simulink model "dbx_control_v1_00"  (R2015a)
settings: Solver=FixedStepDiscrete  SolverMode=SingleTasking  StartTime=0.0  StopTime=20  FixedStep=T_ctrl  RelTol=1e-3
undefined symbols (not defined in the file): A_l_max_x, A_M, A_z_max, CG, epsilon, Flaps_ang_deg, g, h_1, h_2, h_3, Hover_eta_23, Hover_throtle_1, Hover_throtle_23, I_BAC, L_M, m, Roll_pich_sens, Rotation_sign, Servo_calib, T_ctrl, v_i0, Yaw_sens
libraries: DBX_model x29, DBX_Control_lib x22, simulink x10, DBX_Control x3
(part 1 of 3)
settings Model: ExtModeTrigDuration=5000  TunableVars=Flaps_ang_deg,Roll_pich_sens,Throtle_sens,Yaw_sens,p_K_b,p_tau,phi_K_b,phi_f_i,phi_tau,psi_K_b,psi_f_i,psi_tau,q_K_b,q_tau,r_K_b,r_tau,theta_K_b,theta_f_i,theta_tau  TunableVarsStorageClass=Auto,Auto,Auto,Auto,Auto,Auto,Auto,Auto,Auto,Auto,Auto,Auto,Auto,Auto,Auto,Auto,Auto,Auto,Auto  TunableVarsTypeQualifier=,,,,,,,,,,,,,,,,,,  Creator=DavidTorres  LastModifiedBy=David
settings DataIOCC: LimitDataPoints=off  SaveOutput=off  SignalLogging=off  DSMLogging=off  VisualizeSimOutput=off  SaveTime=off
settings OptimizationCC: InlineParams=on  UseDivisionForNetSlopeComputation=on  DefaultUnderspecifiedDataType=single  UseSpecifiedMinMax=on  EfficientFloat2IntCast=on  OptimizeModelRefInitCode=on  MaxStackSize=64  SimCompilerOptimization=on
settings DebuggingCC: SaveWithParameterizedLinksMsg=none  IntegerOverflowMsg=error  StrictBusMsg=ErrorOnBusTreatedAsVector  IntegerSaturationMsg=error
settings HardwareCC: ProdLargestAtomicInteger=Long  ProdLargestAtomicFloat=Double  ProdIntDivRoundTo=Zero  ProdEndianess=LittleEndian  ProdHWDeviceType=Generic->32-bit x86 compatible  TargetLongLongMode=on  TargetIntDivRoundTo=Zero  TargetEndianess=LittleEndian  TargetHWDeviceType=MATLAB Host  ProdEqTarget=off
settings ModelReferenceCC: ModelReferenceNumInstancesAllowed=Single  ModelReferencePassRootInputsByReference=off
settings RTWCC: SystemTargetFile=ert.tlc  GenCodeOnly=on  TemplateMakefile=ert_default_tmf  Description=Embedded Coder  BuildConfiguration=Faster Runs
settings CodeAppCC: IgnoreCustomStorageClasses=off
settings ERTTargetCC: GenerateSampleERTMain=off  ParMdlRefBuildCompliant=on  CompOptLevelCompliant=on  ConcurrentExecutionCompliant=on  ERTFirstTimeCompliant=on  SupportNonFinite=off  SupportComplex=off  SupportContinuousTime=off  ModelStepFunctionPrototypeControlCompliant=on  CPPClassGenCompliant=on  InlinedParameterPlacement=Hierarchical  ERTCustomFileTemplate=example_file_process.tlc

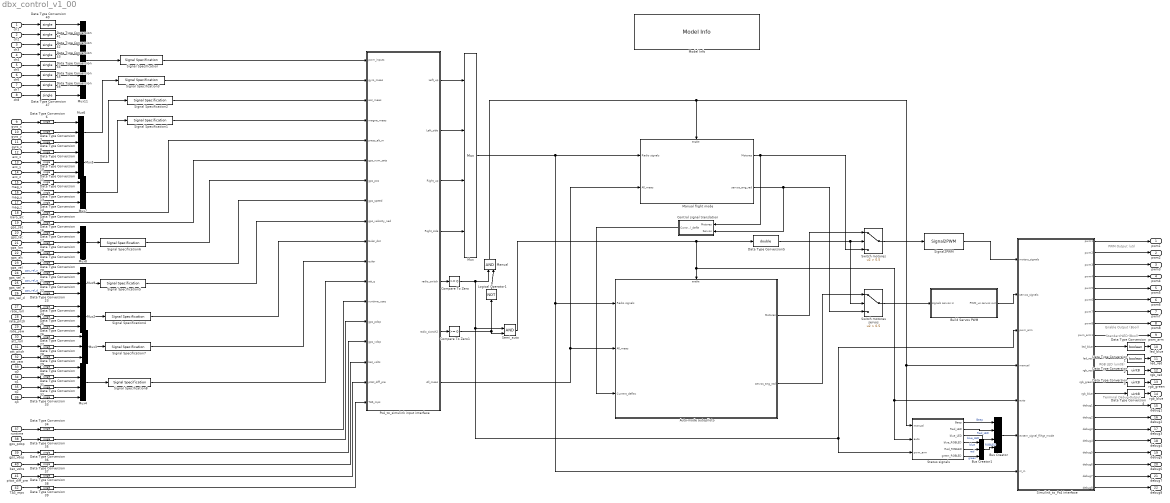
== system dbx_control_v1_00 ==
  note: Terminal Debug Output
  note: RGB LED (uint8)
  note: Standard LED (Bool)
  note: PWM Output (uS)
  note: Enable Output (Bool)
  ch1 : Inport  OutDataTypeStr=double  PortDimensions=[1,1]  SampleTime=T_ctrl
  ch2 : Inport  Port=2  OutDataTypeStr=double  PortDimensions=[1,1]  SampleTime=T_ctrl
  ch3 : Inport  Port=3  OutDataTypeStr=double  PortDimensions=[1,1]  SampleTime=T_ctrl
  ch4 : Inport  Port=4  OutDataTypeStr=double  PortDimensions=[1,1]  SampleTime=T_ctrl
  ch5 : Inport  Port=5  OutDataTypeStr=double  PortDimensions=[1,1]  SampleTime=T_ctrl
  ch6 : Inport  Port=6  OutDataTypeStr=double  PortDimensions=[1,1]  SampleTime=T_ctrl
  ch7 : Inport  Port=7  OutDataTypeStr=double  PortDimensions=[1,1]  SampleTime=T_ctrl
  ch8 : Inport  Port=8  OutDataTypeStr=double  PortDimensions=[1,1]  SampleTime=T_ctrl
  gyro_x : Inport  Port=9  OutDataTypeStr=double  PortDimensions=[1,1]  SampleTime=T_ctrl
  gyro_y : Inport  Port=10  OutDataTypeStr=double  PortDimensions=[1,1]  SampleTime=T_ctrl
  gyro_z : Inport  Port=11  OutDataTypeStr=double  PortDimensions=[1,1]  SampleTime=T_ctrl
  acc_x : Inport  Port=12  OutDataTypeStr=double  PortDimensions=[1,1]  SampleTime=T_ctrl
  acc_y : Inport  Port=13  OutDataTypeStr=double  PortDimensions=[1,1]  SampleTime=T_ctrl
  acc_z : Inport  Port=14  OutDataTypeStr=double  PortDimensions=[1,1]  SampleTime=T_ctrl
  mag_x : Inport  Port=15  OutDataTypeStr=double  PortDimensions=[1,1]  SampleTime=T_ctrl
  mag_y : Inport  Port=16  OutDataTypeStr=double  PortDimensions=[1,1]  SampleTime=T_ctrl
  mag_z : Inport  Port=17  OutDataTypeStr=double  PortDimensions=[1,1]  SampleTime=T_ctrl
  baro_alt : Inport  Port=18  OutDataTypeStr=double  PortDimensions=[1,1]  SampleTime=T_ctrl
  gps_sat : Inport  Port=19  OutDataTypeStr=double  PortDimensions=[1,1]  SampleTime=T_ctrl
  gps_lat : Inport  Port=20  OutDataTypeStr=double  PortDimensions=[1,1]  SampleTime=T_ctrl
  gps_lon : Inport  Port=21  OutDataTypeStr=double  PortDimensions=[1,1]  SampleTime=T_ctrl
  gps_alt : Inport  Port=22  OutDataTypeStr=double  PortDimensions=[1,1]  SampleTime=T_ctrl
  gps_vel : Inport  Port=23  OutDataTypeStr=double  PortDimensions=[1,1]  SampleTime=T_ctrl
  gps_vel_n : Inport  Port=24  OutDataTypeStr=double  PortDimensions=[1,1]  SampleTime=T_ctrl
  gps_vel_e : Inport  Port=25  OutDataTypeStr=double  PortDimensions=[1,1]  SampleTime=T_ctrl
  gps_vel_d : Inport  Port=26  OutDataTypeStr=double  PortDimensions=[1,1]  SampleTime=T_ctrl
  rate_roll : Inport  Port=27  OutDataTypeStr=double  PortDimensions=[1,1]  SampleTime=T_ctrl
  rate_pitch : Inport  Port=28  OutDataTypeStr=double  PortDimensions=[1,1]  SampleTime=T_ctrl
  rate_yaw : Inport  Port=29  OutDataTypeStr=double  PortDimensions=[1,1]  SampleTime=T_ctrl
  att_roll : Inport  Port=30  OutDataTypeStr=double  PortDimensions=[1,1]  SampleTime=T_ctrl
  att_pitch : Inport  Port=31  OutDataTypeStr=double  PortDimensions=[1,1]  SampleTime=T_ctrl
  att_yaw : Inport  Port=32  OutDataTypeStr=double  PortDimensions=[1,1]  SampleTime=T_ctrl
  q0 : Inport  Port=33  OutDataTypeStr=double  PortDimensions=[1,1]  SampleTime=T_ctrl
  q1 : Inport  Port=34  OutDataTypeStr=double  PortDimensions=[1,1]  SampleTime=T_ctrl
  q2 : Inport  Port=35  OutDataTypeStr=double  PortDimensions=[1,1]  SampleTime=T_ctrl
  q3 : Inport  Port=36  OutDataTypeStr=double  PortDimensions=[1,1]  SampleTime=T_ctrl
  runtime : Inport  Port=37  OutDataTypeStr=double  PortDimensions=[1,1]  SampleTime=T_ctrl
  gps_pdop : Inport  Port=38  OutDataTypeStr=double  PortDimensions=[1,1]  SampleTime=T_ctrl
  gps_vdop : Inport  Port=39  OutDataTypeStr=double  PortDimensions=[1,1]  SampleTime=T_ctrl
  bat_volts : Inport  Port=40  OutDataTypeStr=double  PortDimensions=[1,1]  SampleTime=T_ctrl
  pitot_diff_pre : Inport  Port=41  OutDataTypeStr=double  SampleTime=T_ctrl
  TAS_mps : Inport  Port=42  OutDataTypeStr=double  SampleTime=T_ctrl
  Auto-mode autopiloto : Subsystem  TreatAsAtomicUnit=on
  Build Servos PWM : Subsystem  TreatAsAtomicUnit=on
  Bus Creator : BusCreator
  Bus Creator1 : BusCreator  Inputs=3
  Compare To Zero : simulink/Logic and Bit Operations/Compare To Zero  relop=>=  OutDataTypeStr=boolean
  Compare To Zero1 : simulink/Logic and Bit Operations/Compare To Zero  relop=>=  OutDataTypeStr=boolean
  Control signal translation : Subsystem  TreatAsAtomicUnit=on
  Data Type Conversion : DataTypeConversion  OutDataTypeStr=boolean
  Data Type Conversion1 : DataTypeConversion  OutDataTypeStr=boolean
  Data Type Conversion{6..47} (42 alike) : DataTypeConversion  OutDataTypeStr=single
  Data Type Conversion2 : DataTypeConversion  OutDataTypeStr=uint8
  Data Type Conversion3 : DataTypeConversion  OutDataTypeStr=uint8
  Data Type Conversion4 : DataTypeConversion  OutDataTypeStr=uint8
  Data Type Conversion5 : DataTypeConversion  OutDataTypeStr=double
  Logical Operator1 : Logic  Operator=NOT  IconShape=distinctive  AllPortsSameDT=off  OutDataTypeStr=boolean
  Manual : Logic  IconShape=distinctive  AllPortsSameDT=off  OutDataTypeStr=boolean
  Manual flight mode : Subsystem  TreatAsAtomicUnit=on
  Model Info : simulink/Model-Wide Utilities/Model Info  Frame=on  DisplayStringWithTags=|  HorizontalTextAlignment=Center  LeftAlignmentValue=0.5  SourceBlockDiagram=dbx_control_v1_00  TagMaxNumber=20
      | Model Info
      | 
      | Creado por %<Creator>
      | Modificado el %<LastModificationDate> por %<LastModifiedBy>
      | Version %<ModelVersion>
  Mux : Mux
  Mux11 : Mux  Inputs=8
  Mux{2..3,5..9} (7 alike) : Mux  Inputs=3
  Mux4 : Mux
  Px4_to_simulink input interface : Subsystem
  Semi_auto : Logic  IconShape=distinctive  AllPortsSameDT=off  OutDataTypeStr=boolean
  Signal Specification : SignalSpecification  OutDataTypeStr=single  Dimensions=[8,1]
  Signal Specification{1..7} (7 alike) : SignalSpecification  OutDataTypeStr=single  Dimensions=[3,1]
  Signal Specification8 : SignalSpecification  OutDataTypeStr=single  Dimensions=[4,1]
  Signal2PWM : DBX_model/Signal2PWM  b=1  d=0  a=1900  c=1100
  Simulink_to_Px4 interface : Subsystem
  Status signals : Subsystem  TreatAsAtomicUnit=on
  Switch motores : Switch  Criteria=u2 > Threshold  Threshold=0.5
  Switch motores servos : Switch  Criteria=u2 > Threshold  Threshold=0.5
  pwm1 : Outport  PortDimensions=[1,1]
  pwm2 : Outport  Port=2  PortDimensions=[1,1]
  pwm3 : Outport  Port=3  PortDimensions=[1,1]
  pwm4 : Outport  Port=4  PortDimensions=[1,1]
  pwm5 : Outport  Port=5  PortDimensions=[1,1]
  pwm6 : Outport  Port=6  PortDimensions=[1,1]
  pwm7 : Outport  Port=7  PortDimensions=[1,1]
  pwm8 : Outport  Port=8  PortDimensions=[1,1]
  pwm_arm : Outport  Port=9  PortDimensions=[1,1]
  led_blue : Outport  Port=10  OutDataTypeStr=boolean  PortDimensions=[1,1]
  led_red : Outport  Port=11  OutDataTypeStr=boolean  PortDimensions=[1,1]
  rgb_red : Outport  Port=12  OutDataTypeStr=uint8  PortDimensions=[1,1]
  rgb_green : Outport  Port=13  OutDataTypeStr=uint8  PortDimensions=[1,1]
  rgb_blue : Outport  Port=14  OutDataTypeStr=uint8  PortDimensions=[1,1]
  debug1 : Outport  Port=15  PortDimensions=[1,1]
  debug2 : Outport  Port=16  PortDimensions=[1,1]
  debug3 : Outport  Port=17  PortDimensions=[1,1]
  debug4 : Outport  Port=18  PortDimensions=[1,1]
  debug5 : Outport  Port=19  PortDimensions=[1,1]
  debug6 : Outport  Port=20  PortDimensions=[1,1]
  debug7 : Outport  Port=21  PortDimensions=[1,1]
  debug8 : Outport  Port=22  PortDimensions=[1,1]
  wires:
  Switch motores/1 -> Signal2PWM/1
  Switch motores servos/1 -> Build Servos PWM/1(signals servos in)
  Status signals/1(Beep) -> Bus Creator/1  "Beep"
  Status signals/2(Red_LED) -> Bus Creator/2  "Red_LED"
  Status signals/3(blue_LED) -> Bus Creator/3  "blue_LED"
  Status signals/4(blue_RGBLED) -> Bus Creator1/1  "blue"
  Status signals/5(Red_RGBLED) -> Bus Creator1/2  "red"
  Status signals/6(green_RGBLED) -> Bus Creator1/3  "green"
  Bus Creator1/1 -> Bus Creator/4  "RGBLED"
  Simulink_to_Px4 interface/1(pwm1) -> pwm1/1
  Simulink_to_Px4 interface/2(pwm2) -> pwm2/1
  Simulink_to_Px4 interface/3(pwm3) -> pwm3/1
  Simulink_to_Px4 interface/4(pwm4) -> pwm4/1
  Simulink_to_Px4 interface/5(pwm5) -> pwm5/1
  Simulink_to_Px4 interface/6(pwm6) -> pwm6/1
  Simulink_to_Px4 interface/7(pwm7) -> pwm7/1
  Simulink_to_Px4 interface/8(pwm8) -> pwm8/1
  Simulink_to_Px4 interface/10(led_blue) -> Data Type Conversion/1
  Simulink_to_Px4 interface/11(led_red) -> Data Type Conversion1/1
  Simulink_to_Px4 interface/15(debug1) -> debug1/1
  Simulink_to_Px4 interface/17(debug3) -> debug3/1
  Simulink_to_Px4 interface/18(debug4) -> debug4/1
  Simulink_to_Px4 interface/9(pwm_arm1) -> pwm_arm/1
  Simulink_to_Px4 interface/12(rgb_red) -> Data Type Conversion2/1
  Simulink_to_Px4 interface/13(rgb_green) -> Data Type Conversion3/1
  Simulink_to_Px4 interface/14(rgb_blue) -> Data Type Conversion4/1
  Simulink_to_Px4 interface/20(debug6) -> debug6/1
  Simulink_to_Px4 interface/21(debug7) -> debug7/1
  Simulink_to_Px4 interface/22(debug8) -> debug8/1
  Simulink_to_Px4 interface/19(debug5) -> debug5/1
  Data Type Conversion/1 -> led_blue/1
  Data Type Conversion1/1 -> led_red/1
  Data Type Conversion2/1 -> rgb_red/1
  Data Type Conversion3/1 -> rgb_green/1
  Data Type Conversion4/1 -> rgb_blue/1
  Simulink_to_Px4 interface/16(debug2) -> debug2/1
  Signal2PWM/1 -> Simulink_to_Px4 interface/1(motors_signals)
  Build Servos PWM/1(PWM_us servos out) -> Simulink_to_Px4 interface/2(servos_signals)
  Bus Creator/1 -> Simulink_to_Px4 interface/6(extern_signal_flihgt_mode)
  baro_alt/1 -> Data Type Conversion15/1
  gyro_z/1 -> Data Type Conversion8/1
  gyro_y/1 -> Data Type Conversion7/1
  gyro_x/1 -> Data Type Conversion6/1
  acc_z/1 -> Data Type Conversion11/1
  acc_y/1 -> Data Type Conversion10/1
  acc_x/1 -> Data Type Conversion9/1
  mag_x/1 -> Data Type Conversion12/1
  mag_y/1 -> Data Type Conversion13/1
  mag_z/1 -> Data Type Conversion14/1
  ch1/1 -> Data Type Conversion40/1
  ch2/1 -> Data Type Conversion41/1
  ch3/1 -> Data Type Conversion42/1
  ch4/1 -> Data Type Conversion43/1
  ch5/1 -> Data Type Conversion44/1
  ch6/1 -> Data Type Conversion45/1
  runtime/1 -> Data Type Conversion34/1
  ch7/1 -> Data Type Conversion46/1
  ch8/1 -> Data Type Conversion47/1
  att_roll/1 -> Data Type Conversion27/1
  att_pitch/1 -> Data Type Conversion28/1
  att_yaw/1 -> Data Type Conversion29/1
  q0/1 -> Data Type Conversion30/1
  q1/1 -> Data Type Conversion31/1
  q2/1 -> Data Type Conversion32/1
  q3/1 -> Data Type Conversion33/1
  rate_roll/1 -> Data Type Conversion24/1
  rate_pitch/1 -> Data Type Conversion25/1
  rate_yaw/1 -> Data Type Conversion26/1
  gps_vel_n/1 -> Data Type Conversion21/1  "gps_vel_n"
  gps_vel_e/1 -> Data Type Conversion22/1  "gps_vel_e"
  gps_vel_d/1 -> Data Type Conversion23/1  "gps_vel_d"
  gps_lat/1 -> Data Type Conversion17/1
  gps_lon/1 -> Data Type Conversion18/1
  gps_alt/1 -> Data Type Conversion19/1
  gps_vel/1 -> Data Type Conversion20/1
  gps_sat/1 -> Data Type Conversion16/1
  Mux2/1 -> Signal Specification4/1
  Mux3/1 -> Signal Specification7/1
  Mux4/1 -> Signal Specification8/1
  Mux5/1 -> Signal Specification2/1
  Mux6/1 -> Signal Specification3/1
  Mux8/1 -> Signal Specification6/1
  Mux7/1 -> Signal Specification1/1
  Mux11/1 -> Signal Specification/1
  Mux9/1 -> Signal Specification5/1
  gps_pdop/1 -> Data Type Conversion35/1
  gps_vdop/1 -> Data Type Conversion36/1
  bat_volts/1 -> Data Type Conversion37/1
  Signal Specification/1 -> Px4_to_simulink input interface/1(pwm_inputs)
  Signal Specification3/1 -> Px4_to_simulink input interface/2(gyro_meas)
  Signal Specification2/1 -> Px4_to_simulink input interface/3(acc_meas)
  Signal Specification1/1 -> Px4_to_simulink input interface/4(magne_meas)
  Signal Specification6/1 -> Px4_to_simulink input interface/7(gps_pos)
  Signal Specification5/1 -> Px4_to_simulink input interface/9(gps_velocity_ned)
  Signal Specification4/1 -> Px4_to_simulink input interface/10(Euler_dot)
  Signal Specification7/1 -> Px4_to_simulink input interface/11(euler)
  Signal Specification8/1 -> Px4_to_simulink input interface/12(att_q)
  pitot_diff_pre/1 -> Data Type Conversion38/1
  Px4_to_simulink input interface/5(radio_switch) -> Compare To Zero/1
  Px4_to_simulink input interface/6(radio_siwtch2) -> Compare To Zero1/1
  Compare To Zero/1 -> Semi_auto/1, Simulink_to_Px4 interface/3(pwm_arm), Status signals/3(pwm_arm), Manual/1
  Compare To Zero1/1 -> Logical Operator1/1, Semi_auto/2
  Manual/1 -> Simulink_to_Px4 interface/4(manual), Status signals/1(manual), Manual flight mode/Enable
  Manual flight mode/2(servos_ang_rad) -> Control signal translation/2(Servos), Switch motores servos/3
  Auto-mode autopiloto/1(Motores) -> Switch motores/1
  Auto-mode autopiloto/2(servos_ang_rad) -> Switch motores servos/1
  Semi_auto/1 -> Data Type Conversion5/1, Simulink_to_Px4 interface/5(auto), Status signals/2(auto), Auto-mode autopiloto/Enable
  Data Type Conversion5/1 -> Switch motores servos/2, Switch motores/2
  Px4_to_simulink input interface/4(Right_side) -> Mux/4
  Px4_to_simulink input interface/3(Right_up) -> Mux/3
  Px4_to_simulink input interface/2(Left_side) -> Mux/2
  Px4_to_simulink input interface/1(Left_up) -> Mux/1
  Px4_to_simulink input interface/7(All_meas) -> Manual flight mode/2(All_meas), Auto-mode autopiloto/2(All_meas)
  Mux/1 -> Manual flight mode/1(Radio signals), Simulink_to_Px4 interface/7(rc_in), Auto-mode autopiloto/1(Radio signals)
  TAS_mps/1 -> Data Type Conversion39/1
  Logical Operator1/1 -> Manual/2
  Manual flight mode/1(Motores) -> Switch motores/3, Control signal translation/1(Motores)
  Control signal translation/1(Control_defle) -> Auto-mode autopiloto/3(Current_deflex)
  Data Type Conversion6/1 -> Mux6/1
  Data Type Conversion7/1 -> Mux6/2
  Data Type Conversion8/1 -> Mux6/3
  Data Type Conversion9/1 -> Mux5/1
  Data Type Conversion10/1 -> Mux5/2
  Data Type Conversion11/1 -> Mux5/3
  Data Type Conversion12/1 -> Mux7/1
  Data Type Conversion13/1 -> Mux7/2
  Data Type Conversion14/1 -> Mux7/3
  Data Type Conversion15/1 -> Px4_to_simulink input interface/5(press_alt_m)
  Data Type Conversion16/1 -> Px4_to_simulink input interface/6(gps_num_sats)
  Data Type Conversion17/1 -> Mux8/1
  Data Type Conversion18/1 -> Mux8/2
  Data Type Conversion19/1 -> Mux8/3
  Data Type Conversion20/1 -> Px4_to_simulink input interface/8(gps_speed)
  Data Type Conversion21/1 -> Mux9/1
  Data Type Conversion22/1 -> Mux9/2
  Data Type Conversion23/1 -> Mux9/3
  Data Type Conversion24/1 -> Mux2/1
  Data Type Conversion25/1 -> Mux2/2
  Data Type Conversion26/1 -> Mux2/3
  Data Type Conversion27/1 -> Mux3/1
  Data Type Conversion28/1 -> Mux3/2
  Data Type Conversion29/1 -> Mux3/3
  Data Type Conversion30/1 -> Mux4/1
  Data Type Conversion31/1 -> Mux4/2
  Data Type Conversion32/1 -> Mux4/3
  Data Type Conversion33/1 -> Mux4/4
  Data Type Conversion34/1 -> Px4_to_simulink input interface/13(runtime_usec)
  Data Type Conversion35/1 -> Px4_to_simulink input interface/14(gps_pdop)
  Data Type Conversion36/1 -> Px4_to_simulink input interface/15(gps_vdop)
  Data Type Conversion37/1 -> Px4_to_simulink input interface/16(bat_volts)
  Data Type Conversion38/1 -> Px4_to_simulink input interface/17(pitot_diff_pre)
  Data Type Conversion39/1 -> Px4_to_simulink input interface/18(TAS_mps)
  Data Type Conversion40/1 -> Mux11/1
  Data Type Conversion41/1 -> Mux11/2
  Data Type Conversion42/1 -> Mux11/3
  Data Type Conversion43/1 -> Mux11/4
  Data Type Conversion44/1 -> Mux11/5
  Data Type Conversion45/1 -> Mux11/6
  Data Type Conversion46/1 -> Mux11/7
  Data Type Conversion47/1 -> Mux11/8

== system dbx_control_v1_00/Auto-mode autopiloto ==
  Radio signals : Inport
  All_meas : Inport  Port=2
  Current_deflex : Inport  Port=3
  Enable : EnablePort  ShowOutputPort=on
  Activation bus : Subsystem  TreatAsAtomicUnit=on
  DBX advance control system : Subsystem
  Demux : Demux  Outputs=7
  Ground : Ground
  Ground1 : Ground
  Initial conditions : Subsystem  TreatAsAtomicUnit=on
  Mux : Mux  Inputs=3
  Mux1 : Mux  Inputs=7
  Mux2 : Mux  Inputs=3
  Saturation : Saturate  UpperLimit=1  LowerLimit=0
  Saturation1 : Saturate  UpperLimit=deg2rad(90)  LowerLimit=-deg2rad(90)
  Sensibilidades Radio : Subsystem  TreatAsAtomicUnit=on
  Sup2Servo Lin conversion : DBX_model/Sup2Servo Lin conversion  Gain=Servo_calib.Servo1.Pendiente_Sup_Servo  Bias=Servo_calib.Servo1.Sup_rad_0
  Sup2Servo Lin conversion1 : DBX_model/Sup2Servo Lin conversion  Gain=Servo_calib.Servo2.Pendiente_Sup_Servo  Bias=Servo_calib.Servo2.Sup_rad_0
  Sup2Servo Lin conversion2 : DBX_model/Sup2Servo Lin conversion  Gain=Servo_calib.Servo3.Pendiente_Sup_Servo  Bias=Servo_calib.Servo3.Sup_rad_0
  Sup2Servo Lin conversion3 : DBX_model/Sup2Servo Lin conversion  Gain=Servo_calib.Servo4.Pendiente_Sup_Servo  Bias=Servo_calib.Servo4.Sup_rad_0
  Sup2Servo Lin conversion4 : DBX_model/Sup2Servo Lin conversion  Gain=Servo_calib.Servo5.Pendiente_Sup_Servo  Bias=Servo_calib.Servo5.Sup_rad_0
  Sup2Servo Lin conversion5 : DBX_model/Sup2Servo Lin conversion  Gain=Servo_calib.Servo6.Pendiente_Sup_Servo  Bias=Servo_calib.Servo6.Sup_rad_0
  Sup2Servo Lin conversion6 : DBX_model/Sup2Servo Lin conversion  Gain=Servo_calib.Servo7.Pendiente_Sup_Servo  Bias=Servo_calib.Servo7.Sup_rad_0
  Terminator : Terminator
  Motores : Outport
  servos_ang_rad : Outport  Port=2
  wires:
  DBX advance control system/1(Mot_throtles) -> Saturation/1
  Saturation/1 -> Motores/1
  Mux1/1 -> Saturation1/1
  Saturation1/1 -> servos_ang_rad/1
  Sup2Servo Lin conversion/1 -> Mux1/1
  Sup2Servo Lin conversion1/1 -> Mux1/2
  Sup2Servo Lin conversion2/1 -> Mux1/3
  Sup2Servo Lin conversion3/1 -> Mux1/4
  Sup2Servo Lin conversion4/1 -> Mux1/5
  Sup2Servo Lin conversion5/1 -> Mux1/6
  Sup2Servo Lin conversion6/1 -> Mux1/7
  All_meas/1 -> Initial conditions/1(All_meas), DBX advance control system/5(All_meas)
  DBX advance control system/3(surf_angles) -> Demux/1
  Demux/1 -> Sup2Servo Lin conversion/1
  Demux/2 -> Sup2Servo Lin conversion1/1
  Demux/3 -> Sup2Servo Lin conversion2/1
  Demux/4 -> Sup2Servo Lin conversion3/1
  Demux/5 -> Sup2Servo Lin conversion4/1
  Demux/6 -> Sup2Servo Lin conversion5/1
  Demux/7 -> Sup2Servo Lin conversion6/1
  Radio signals/1 -> Sensibilidades Radio/1(Radio_in)
  Mux/1 -> DBX advance control system/3(Att_ref(rad))
  Mux2/1 -> DBX advance control system/1(Vel_ref_yaw(mps))
  Sensibilidades Radio/4(Yaw(radps)) -> DBX advance control system/4(Yaw_rate_ref(rad)), Mux/3
  Sensibilidades Radio/2(Roll(rad)) -> Mux/1
  Sensibilidades Radio/3(Vx_yaw) -> Mux2/1
  Activation bus/1(Activation bus) -> DBX advance control system/8(activation_bus)
  Enable/1 -> DBX advance control system/9(Int_reset), Activation bus/2(Activation1), Activation bus/1(Activation), Activation bus/4(Activation3), Activation bus/3(Activation2)
  Initial conditions/1(Init_cond) -> DBX advance control system/6(Init_cond)
  Current_deflex/1 -> DBX advance control system/7(Init_deflect)
  DBX advance control system/2(Control_signals) -> Terminator/1
  Ground/1 -> Mux2/3, Mux2/2
  Ground1/1 -> Mux/2
  Sensibilidades Radio/1(accz_yaw) -> DBX advance control system/2(Acc_z(mps2))

== system dbx_control_v1_00/Build Servos PWM ==
  note: Estos 4 ultimos significa que
      | los ejes de los servos deben
      | apuntar el la direccion +y
  note: Control input
      | Rango
      | Direccion rot/Dir servos
      | Rango del servo
      |
      | eta_1 (rad) (Pan arm 1)
      | -90,90
      | -1
      | 180
      |
      | eta_2 (rad) (Pan arm 2
      | -90,90
      | -1
      | 180
      |
      | eta_3 (rad) (Pan arm 3)
      | -90,90
      | 1
      | 180
      |
      | Rudervator Left (rad)
      | -90,90
      | 1
      | 180
      |
      | Rudervator Right (rad)
      | -90,90
      | 1
      | 180
      |
      | Aileron Left (rad)
      | -90,90
      | 1
      | 180
      |
      | Aielron Right (rad)
      | -90,90
      | 1
      | 180
  signals servos in : Inport
  Demux : Demux  Outputs=7
  Mux : Mux  Inputs=7
  Signal2PWM{,1..6} (7 alike) : DBX_model/Signal2PWM  b=deg2rad(90)  d=-deg2rad(90)  a=1900  c=1100
  PWM_us servos out : Outport
  wires:
  Mux/1 -> PWM_us servos out/1
  signals servos in/1 -> Demux/1
  Demux/6 -> Signal2PWM5/1
  Demux/5 -> Signal2PWM4/1
  Demux/4 -> Signal2PWM3/1
  Demux/3 -> Signal2PWM2/1
  Demux/2 -> Signal2PWM1/1
  Demux/1 -> Signal2PWM/1
  Signal2PWM/1 -> Mux/1
  Signal2PWM1/1 -> Mux/2
  Signal2PWM3/1 -> Mux/4
  Signal2PWM4/1 -> Mux/5
  Signal2PWM2/1 -> Mux/3
  Signal2PWM5/1 -> Mux/6
  Demux/7 -> Signal2PWM6/1
  Signal2PWM6/1 -> Mux/7

== system dbx_control_v1_00/Control signal translation ==
  Motores : Inport
  Servos : Inport  Port=2
  Demux : Demux  Outputs=3
  Ground{,1..4} (5 alike) : Ground
  Mux1 : Mux  Inputs=9
  Selector : Selector  InputPortWidth=7  Indices=3
  Servo2Sup Lin conversion : DBX_model/Servo2Sup Lin conversion  Gain=Servo_calib.Servo3.Pendiente_Sup_Servo  Bias=Servo_calib.Servo3.Sup_rad_0
  Control_defle : Outport
  wires:
  Mux1/1 -> Control_defle/1
  Demux/1 -> Mux1/1
  Servos/1 -> Selector/1
  Demux/2 -> Mux1/3
  Demux/3 -> Mux1/5
  Ground/1 -> Mux1/2
  Ground1/1 -> Mux1/4
  Ground2/1 -> Mux1/7
  Ground3/1 -> Mux1/8
  Ground4/1 -> Mux1/9
  Servo2Sup Lin conversion/1 -> Mux1/6
  Motores/1 -> Demux/1
  Selector/1 -> Servo2Sup Lin conversion/1

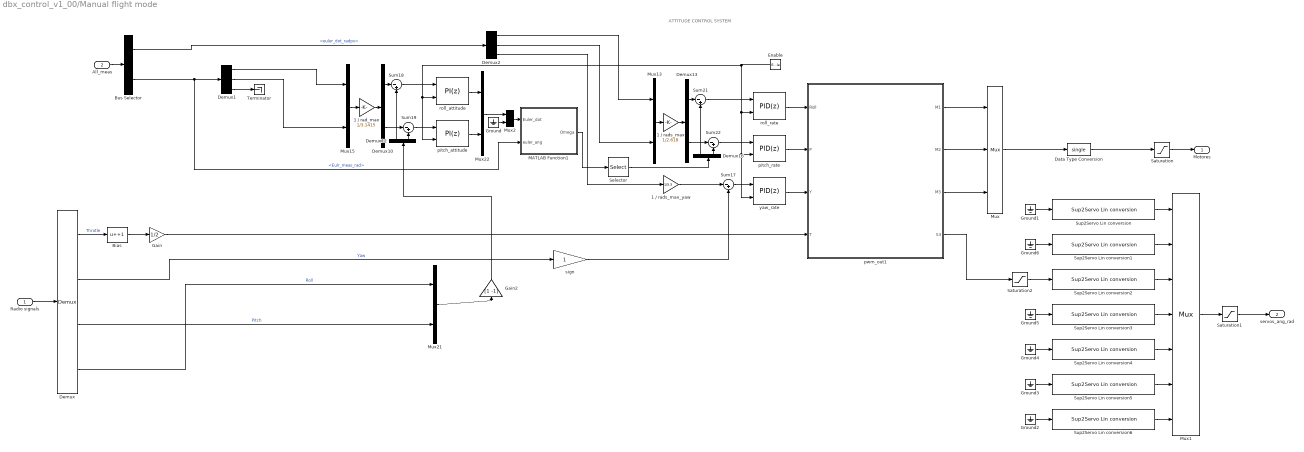
== system dbx_control_v1_00/Manual flight mode ==
  note: ATTITUDE CONTROL SYSTEM
  Radio signals : Inport
  All_meas : Inport  Port=2
  Enable : EnablePort  ShowOutputPort=on
  1 / rad_max : Gain  Gain=1/3.1415
  1 / rads_max : Gain  Gain=1/2.618
  1 / rads_max_yaw : Gain  Gain=1/5.3
  Bias : Bias  Bias=+1
  Bus Selector : BusSelector  OutputSignals=Meas.euler_dot_radps,Meas.Eulr_meas_rad
  Data Type Conversion : DataTypeConversion  OutDataTypeStr=single
  Demux : Demux
  Demux1 : Demux  Outputs=3
  Demux{10,12..13,16} (4 alike) : Demux  Outputs=2
  Demux2 : Demux  Outputs=3
  Gain : Gain  Gain=1/2
  Gain2 : Gain  Gain=[1 -1]
  Ground{,1..6} (7 alike) : Ground
  MATLAB Function1 : MATLAB Function  TreatAsAtomicUnit=on
  Mux : Mux  Inputs=3
  Mux1 : Mux  Inputs=7
  Mux{13,15,21..22} (4 alike) : Mux  Inputs=2
  Mux2 : Mux  Inputs=[2,1]
  Saturation : Saturate  UpperLimit=1  LowerLimit=0
  Saturation1 : Saturate  UpperLimit=deg2rad(90)  LowerLimit=-deg2rad(90)  OutDataTypeStr=single
  Saturation2 : Saturate  UpperLimit=deg2rad(20)  LowerLimit=-deg2rad(20)
  Selector : Selector  InputPortWidth=3  Indices=[1:2]
  Sum{17..19,21..22} (5 alike) : Sum  Inputs=|-+
  Sup2Servo Lin conversion : DBX_model/Sup2Servo Lin conversion  Gain=Servo_calib.Servo1.Pendiente_Sup_Servo  Bias=Servo_calib.Servo1.Sup_rad_0
  Sup2Servo Lin conversion1 : DBX_model/Sup2Servo Lin conversion  Gain=Servo_calib.Servo2.Pendiente_Sup_Servo  Bias=Servo_calib.Servo2.Sup_rad_0
  Sup2Servo Lin conversion2 : DBX_model/Sup2Servo Lin conversion  Gain=Servo_calib.Servo3.Pendiente_Sup_Servo  Bias=Servo_calib.Servo3.Sup_rad_0
  Sup2Servo Lin conversion3 : DBX_model/Sup2Servo Lin conversion  Gain=Servo_calib.Servo4.Pendiente_Sup_Servo  Bias=Servo_calib.Servo4.Sup_rad_0
  Sup2Servo Lin conversion4 : DBX_model/Sup2Servo Lin conversion  Gain=Servo_calib.Servo5.Pendiente_Sup_Servo  Bias=Servo_calib.Servo5.Sup_rad_0
  Sup2Servo Lin conversion5 : DBX_model/Sup2Servo Lin conversion  Gain=Servo_calib.Servo6.Pendiente_Sup_Servo  Bias=Servo_calib.Servo6.Sup_rad_0
  Sup2Servo Lin conversion6 : DBX_model/Sup2Servo Lin conversion  Gain=Servo_calib.Servo7.Pendiente_Sup_Servo  Bias=Servo_calib.Servo7.Sup_rad_0
  Terminator : Terminator
  pitch_attitude : simulink/Continuous/PID Controller  Controller=PI  TimeDomain=Discrete-time  SampleTime=-1  IntegratorMethod=Forward Euler  FilterMethod=Forward Euler  Form=Parallel  UseFilter=on  ControllerParametersSource=internal  P=0.5  I=0.1  D=0  N=100  InitialConditionSource=internal  InitialConditionForIntegrator=0  InitialConditionForFilter=0  ExternalReset=either  LimitOutput=on  UpperSaturationLimit=1  LowerSaturationLimit=-1  LinearizeAsGain=on  AntiWindupMode=none  Kb=1  TrackingMode=off  Kt=1  PParamMin=[]  PParamMax=[]  IParamMin=[]  IParamMax=[]  DParamMin=[]  DParamMax=[]  NParamMin=[]  NParamMax=[]  KbParamMin=[]  KbParamMax=[]  KtParamMin=[]  KtParamMax=[]  POutMin=[]  POutMax=[]  IOutMin=[]  IOutMax=[]  DOutMin=[]  DOutMax=[]  NOutMin=[]  NOutMax=[]  KbOutMin=[]  KbOutMax=[]  KtOutMin=[]  KtOutMax=[]  IntegratorOutMin=[]  IntegratorOutMax=[]  FilterOutMin=[]  FilterOutMax=[]  SumOutMin=[]  SumOutMax=[]  SumI1OutMin=[]  SumI1OutMax=[]  SumI2OutMin=[]  SumI2OutMax=[]  SumI3OutMin=[]  SumI3OutMax=[]  SumDOutMin=[]  SumDOutMax=[]  SaturationOutMin=[]  SaturationOutMax=[]  IntegratorContinuousStateAttributes=''  IntegratorStateMustResolveToSignalObject=off  IntegratorRTWStateStorageClass=Auto  FilterContinuousStateAttributes=''  FilterStateMustResolveToSignalObject=off  FilterRTWStateStorageClass=Auto  DifferentiatorICPrevScaledInput=0  DifferentiatorOutMin=[]  DifferentiatorOutMax=[]
  pitch_rate : simulink/Continuous/PID Controller  Controller=PID  TimeDomain=Discrete-time  SampleTime=-1  IntegratorMethod=Forward Euler  FilterMethod=Forward Euler  Form=Parallel  UseFilter=on  ControllerParametersSource=internal  P=1  I=0  D=0  N=100  InitialConditionSource=internal  InitialConditionForIntegrator=0  InitialConditionForFilter=0  ExternalReset=either  LimitOutput=on  UpperSaturationLimit=1  LowerSaturationLimit=-1  LinearizeAsGain=on  AntiWindupMode=none  Kb=1  TrackingMode=off  Kt=1  PParamMin=[]  PParamMax=[]  IParamMin=[]  IParamMax=[]  DParamMin=[]  DParamMax=[]  NParamMin=[]  NParamMax=[]  KbParamMin=[]  KbParamMax=[]  KtParamMin=[]  KtParamMax=[]  POutMin=[]  POutMax=[]  IOutMin=[]  IOutMax=[]  DOutMin=[]  DOutMax=[]  NOutMin=[]  NOutMax=[]  KbOutMin=[]  KbOutMax=[]  KtOutMin=[]  KtOutMax=[]  IntegratorOutMin=[]  IntegratorOutMax=[]  FilterOutMin=[]  FilterOutMax=[]  SumOutMin=[]  SumOutMax=[]  SumI1OutMin=[]  SumI1OutMax=[]  SumI2OutMin=[]  SumI2OutMax=[]  SumI3OutMin=[]  SumI3OutMax=[]  SumDOutMin=[]  SumDOutMax=[]  SaturationOutMin=[]  SaturationOutMax=[]  IntegratorContinuousStateAttributes=''  IntegratorStateMustResolveToSignalObject=off  IntegratorRTWStateStorageClass=Auto  FilterContinuousStateAttributes=''  FilterStateMustResolveToSignalObject=off  FilterRTWStateStorageClass=Auto  DifferentiatorICPrevScaledInput=0  DifferentiatorOutMin=[]  DifferentiatorOutMax=[]
  pwm_out1 : MATLAB Function  TreatAsAtomicUnit=on  SystemSampleTime=T_ctrl
  roll_attitude : simulink/Continuous/PID Controller  Controller=PI  TimeDomain=Discrete-time  SampleTime=-1  IntegratorMethod=Forward Euler  FilterMethod=Forward Euler  Form=Parallel  UseFilter=on  ControllerParametersSource=internal  P=0.5  I=0.1  D=0  N=100  InitialConditionSource=internal  InitialConditionForIntegrator=0  InitialConditionForFilter=0  ExternalReset=either  LimitOutput=on  UpperSaturationLimit=1  LowerSaturationLimit=-1  LinearizeAsGain=on  AntiWindupMode=none  Kb=1  TrackingMode=off  Kt=1  PParamMin=[]  PParamMax=[]  IParamMin=[]  IParamMax=[]  DParamMin=[]  DParamMax=[]  NParamMin=[]  NParamMax=[]  KbParamMin=[]  KbParamMax=[]  KtParamMin=[]  KtParamMax=[]  POutMin=[]  POutMax=[]  IOutMin=[]  IOutMax=[]  DOutMin=[]  DOutMax=[]  NOutMin=[]  NOutMax=[]  KbOutMin=[]  KbOutMax=[]  KtOutMin=[]  KtOutMax=[]  IntegratorOutMin=[]  IntegratorOutMax=[]  FilterOutMin=[]  FilterOutMax=[]  SumOutMin=[]  SumOutMax=[]  SumI1OutMin=[]  SumI1OutMax=[]  SumI2OutMin=[]  SumI2OutMax=[]  SumI3OutMin=[]  SumI3OutMax=[]  SumDOutMin=[]  SumDOutMax=[]  SaturationOutMin=[]  SaturationOutMax=[]  IntegratorContinuousStateAttributes=''  IntegratorStateMustResolveToSignalObject=off  IntegratorRTWStateStorageClass=Auto  FilterContinuousStateAttributes=''  FilterStateMustResolveToSignalObject=off  FilterRTWStateStorageClass=Auto  DifferentiatorICPrevScaledInput=0  DifferentiatorOutMin=[]  DifferentiatorOutMax=[]
  roll_rate : simulink/Continuous/PID Controller  Controller=PID  TimeDomain=Discrete-time  SampleTime=-1  IntegratorMethod=Forward Euler  FilterMethod=Forward Euler  Form=Parallel  UseFilter=on  ControllerParametersSource=internal  P=1  I=0  D=0  N=100  InitialConditionSource=internal  InitialConditionForIntegrator=0  InitialConditionForFilter=0  ExternalReset=either  LimitOutput=on  UpperSaturationLimit=1  LowerSaturationLimit=-1  LinearizeAsGain=on  AntiWindupMode=none  Kb=1  TrackingMode=off  Kt=1  PParamMin=[]  PParamMax=[]  IParamMin=[]  IParamMax=[]  DParamMin=[]  DParamMax=[]  NParamMin=[]  NParamMax=[]  KbParamMin=[]  KbParamMax=[]  KtParamMin=[]  KtParamMax=[]  POutMin=[]  POutMax=[]  IOutMin=[]  IOutMax=[]  DOutMin=[]  DOutMax=[]  NOutMin=[]  NOutMax=[]  KbOutMin=[]  KbOutMax=[]  KtOutMin=[]  KtOutMax=[]  IntegratorOutMin=[]  IntegratorOutMax=[]  FilterOutMin=[]  FilterOutMax=[]  SumOutMin=[]  SumOutMax=[]  SumI1OutMin=[]  SumI1OutMax=[]  SumI2OutMin=[]  SumI2OutMax=[]  SumI3OutMin=[]  SumI3OutMax=[]  SumDOutMin=[]  SumDOutMax=[]  SaturationOutMin=[]  SaturationOutMax=[]  IntegratorContinuousStateAttributes=''  IntegratorStateMustResolveToSignalObject=off  IntegratorRTWStateStorageClass=Auto  FilterContinuousStateAttributes=''  FilterStateMustResolveToSignalObject=off  FilterRTWStateStorageClass=Auto  DifferentiatorICPrevScaledInput=0  DifferentiatorOutMin=[]  DifferentiatorOutMax=[]
  sign : Gain
  yaw_rate : simulink/Continuous/PID Controller  Controller=PID  TimeDomain=Discrete-time  SampleTime=-1  IntegratorMethod=Forward Euler  FilterMethod=Forward Euler  Form=Parallel  UseFilter=on  ControllerParametersSource=internal  P=2  I=0.2  D=0  N=100  InitialConditionSource=internal  InitialConditionForIntegrator=0  InitialConditionForFilter=0  ExternalReset=either  LimitOutput=on  UpperSaturationLimit=1  LowerSaturationLimit=-1  LinearizeAsGain=on  AntiWindupMode=none  Kb=1  TrackingMode=off  Kt=1  PParamMin=[]  PParamMax=[]  IParamMin=[]  IParamMax=[]  DParamMin=[]  DParamMax=[]  NParamMin=[]  NParamMax=[]  KbParamMin=[]  KbParamMax=[]  KtParamMin=[]  KtParamMax=[]  POutMin=[]  POutMax=[]  IOutMin=[]  IOutMax=[]  DOutMin=[]  DOutMax=[]  NOutMin=[]  NOutMax=[]  KbOutMin=[]  KbOutMax=[]  KtOutMin=[]  KtOutMax=[]  IntegratorOutMin=[]  IntegratorOutMax=[]  FilterOutMin=[]  FilterOutMax=[]  SumOutMin=[]  SumOutMax=[]  SumI1OutMin=[]  SumI1OutMax=[]  SumI2OutMin=[]  SumI2OutMax=[]  SumI3OutMin=[]  SumI3OutMax=[]  SumDOutMin=[]  SumDOutMax=[]  SaturationOutMin=[]  SaturationOutMax=[]  IntegratorContinuousStateAttributes=''  IntegratorStateMustResolveToSignalObject=off  IntegratorRTWStateStorageClass=Auto  FilterContinuousStateAttributes=''  FilterStateMustResolveToSignalObject=off  FilterRTWStateStorageClass=Auto  DifferentiatorICPrevScaledInput=0  DifferentiatorOutMin=[]  DifferentiatorOutMax=[]
  Motores : Outport
  servos_ang_rad : Outport  Port=2
  wires:
  Radio signals/1 -> Demux/1
  Mux/1 -> Data Type Conversion/1
  Saturation/1 -> Motores/1
  Demux/1 -> Bias/1  "Throtle"
  Bias/1 -> Gain/1
  Demux/2 -> sign/1  "Yaw"
  Demux/3 -> Mux21/2  "Pitch"
  Demux/4 -> Mux21/1  "Roll"
  Mux1/1 -> Saturation1/1
  Saturation1/1 -> servos_ang_rad/1
  Sup2Servo Lin conversion/1 -> Mux1/1
  Sup2Servo Lin conversion1/1 -> Mux1/2
  Sup2Servo Lin conversion2/1 -> Mux1/3
  Ground2/1 -> Sup2Servo Lin conversion6/1
  Ground3/1 -> Sup2Servo Lin conversion5/1
  Ground4/1 -> Sup2Servo Lin conversion4/1
  Ground5/1 -> Sup2Servo Lin conversion3/1
  Sup2Servo Lin conversion3/1 -> Mux1/4
  Sup2Servo Lin conversion4/1 -> Mux1/5
  Sup2Servo Lin conversion5/1 -> Mux1/6
  Sup2Servo Lin conversion6/1 -> Mux1/7
  Sum21/1 -> roll_rate/1
  1 / rads_max/1 -> Demux13/1
  Demux13/2 -> Sum22/1
  Demux13/1 -> Sum21/1
  Sum17/1 -> yaw_rate/1
  Sum22/1 -> pitch_rate/1
  Mux13/1 -> 1 / rads_max/1
  pitch_rate/1 -> pwm_out1/2(P)
  Sum18/1 -> roll_attitude/1
  1 / rad_max/1 -> Demux10/1
  Demux10/2 -> Sum19/1
  Demux10/1 -> Sum18/1
  Demux2/1 -> Mux13/1
  Demux12/2 -> Sum19/2
  Demux12/1 -> Sum18/2
  Demux16/2 -> Sum22/2
  Demux16/1 -> Sum21/2
  roll_attitude/1 -> Mux22/1
  pitch_attitude/1 -> Mux22/2
  Demux2/3 -> 1 / rads_max_yaw/1
  Demux2/2 -> Mux13/2
  Sum19/1 -> pitch_attitude/1
  roll_rate/1 -> pwm_out1/1(Roll)
  1 / rads_max_yaw/1 -> Sum17/1
  Mux21/1 -> Gain2/1
  Demux1/2 -> Mux15/2
  Mux15/1 -> 1 / rad_max/1
  Demux1/1 -> Mux15/1
  yaw_rate/1 -> pwm_out1/3(Y)
  Gain2/1 -> Demux12/1
  Enable/1 -> pitch_attitude/2, roll_attitude/2, yaw_rate/2, pitch_rate/2, roll_rate/2
  Ground1/1 -> Sup2Servo Lin conversion/1
  Ground6/1 -> Sup2Servo Lin conversion1/1
  pwm_out1/4(S3) -> Saturation2/1
  pwm_out1/1(M1) -> Mux/1
  pwm_out1/2(M2) -> Mux/2
  pwm_out1/3(M3) -> Mux/3
  Saturation2/1 -> Sup2Servo Lin conversion2/1
  sign/1 -> Sum17/2
  All_meas/1 -> Bus Selector/1
  Bus Selector/2 -> MATLAB Function1/2(euler_ang), Demux1/1  "<Eulr_meas_rad>"
  Bus Selector/1 -> Demux2/1  "<euler_dot_radps>"
  Demux1/3 -> Terminator/1
  Gain/1 -> pwm_out1/4(T)
  Data Type Conversion/1 -> Saturation/1
  Mux22/1 -> Mux2/1
  Mux2/1 -> MATLAB Function1/1(Euler_dot)
  Ground/1 -> Mux2/2
  Selector/1 -> Demux16/1
  MATLAB Function1/1(Omega) -> Selector/1

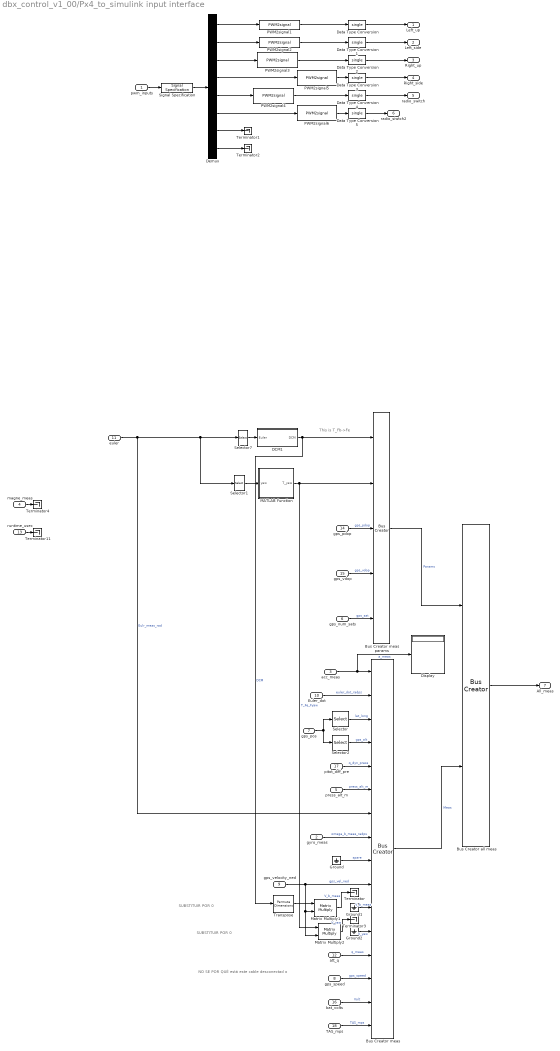
== system dbx_control_v1_00/Px4_to_simulink input interface ==
  note: NO SE POR QUÉ está este cable desconectad o
  note: SUBSTITUIR POR 0
  note: This is T_Fb->Fe
  note: SUBSTITUIR POR 0
  pwm_inputs : Inport  PortDimensions=8  SampleTime=T_ctrl
  gyro_meas : Inport  Port=2  PortDimensions=3  SampleTime=T_ctrl
  acc_meas : Inport  Port=3  PortDimensions=3  SampleTime=T_ctrl
  magne_meas : Inport  Port=4  PortDimensions=3  SampleTime=T_ctrl
  press_alt_m : Inport  Port=5  PortDimensions=1  SampleTime=T_ctrl
  gps_num_sats : Inport  Port=6  PortDimensions=1  SampleTime=T_ctrl
  gps_pos : Inport  Port=7  PortDimensions=3  SampleTime=T_ctrl
  gps_speed : Inport  Port=8  PortDimensions=1  SampleTime=T_ctrl
  gps_velocity_ned : Inport  Port=9  PortDimensions=3  SampleTime=T_ctrl
  Euler_dot : Inport  Port=10  PortDimensions=3  SampleTime=T_ctrl
  euler : Inport  Port=11  PortDimensions=3  SampleTime=T_ctrl
  att_q : Inport  Port=12  PortDimensions=4  SampleTime=T_ctrl
  runtime_usec : Inport  Port=13  PortDimensions=1  SampleTime=T_ctrl
  gps_pdop : Inport  Port=14  PortDimensions=1  SampleTime=T_ctrl
  gps_vdop : Inport  Port=15  PortDimensions=1  SampleTime=T_ctrl
  bat_volts : Inport  Port=16  PortDimensions=1  SampleTime=T_ctrl
  pitot_diff_pre : Inport  Port=17  SampleTime=T_ctrl
  TAS_mps : Inport  Port=18  SampleTime=T_ctrl
  Bus Creator all meas : BusCreator  Inputs=2
  Bus Creator meas : BusCreator  Inputs=16
  Bus Creator meas params : BusCreator  Inputs=5
  DCM1 : Subsystem  TreatAsAtomicUnit=on
  Data Type Conversion{,1..5} (6 alike) : DataTypeConversion  OutDataTypeStr=single
  Demux : Demux  Outputs=8
  Display : Display
  Ground : Ground
  Ground1 : Ground
  Ground2 : Ground
  MATLAB Function : MATLAB Function  TreatAsAtomicUnit=on
  Matrix Multiply1 : Product  Multiplication=Matrix(*)
  Matrix Multiply2 : Product  Multiplication=Matrix(*)
  PWM2signal{1..6} (6 alike) : DBX_model/PWM2signal  c=2000  a=1000  d=1  b=-1
  Selector : Selector  InputPortWidth=3  Indices=[1,2]
  Selector1 : Selector  InputPortWidth=3  Indices=3
  Selector2 : Selector  InputPortWidth=3  Indices=3
  Selector7 : Selector  InputPortWidth=3  Indices=[3 2 1]
  Signal Specification : SignalSpecification  Dimensions=8
  Terminator{,1..4,11} (6 alike) : Terminator
  Transpose : PermuteDimensions
  Left_up : Outport
  Left_side : Outport  Port=2
  Right_up : Outport  Port=3
  Right_side : Outport  Port=4
  radio_switch : Outport  Port=5
  radio_siwtch2 : Outport  Port=6
  All_meas : Outport  Port=7
  wires:
  PWM2signal1/1 -> Data Type Conversion/1
  PWM2signal2/1 -> Data Type Conversion1/1
  PWM2signal3/1 -> Data Type Conversion2/1
  PWM2signal5/1 -> Data Type Conversion3/1
  Bus Creator all meas/1 -> All_meas/1
  PWM2signal4/1 -> Data Type Conversion4/1
  att_q/1 -> Bus Creator meas/13  "q_meas"
  euler/1 -> Bus Creator meas/7, Selector1/1, Selector7/1  "Eulr_meas_rad"
  Euler_dot/1 -> Bus Creator meas/2  "euler_dot_radps"
  bat_volts/1 -> Bus Creator meas/15  "Volt"
  Bus Creator meas/1 -> Bus Creator all meas/2  "Meas"
  Bus Creator meas params/1 -> Bus Creator all meas/1  "Params"
  DCM1/1(DCM) -> Transpose/1, Bus Creator meas params/1  "DCM"
  acc_meas/1 -> Display/1, Bus Creator meas/1  "a_meas"
  gps_pdop/1 -> Bus Creator meas params/3  "gps_pdop"
  gps_num_sats/1 -> Bus Creator meas params/5  "gps_sat"
  gps_vdop/1 -> Bus Creator meas params/4  "gps_vdop"
  Selector7/1 -> DCM1/1(Euler)
  Selector1/1 -> MATLAB Function/1(yaw)
  MATLAB Function/1(T_yaw) -> Matrix Multiply2/1, Bus Creator meas params/2  "T_Fe_Fyaw"
  Demux/1 -> PWM2signal1/1
  Demux/2 -> PWM2signal2/1
  Demux/3 -> PWM2signal3/1
  Demux/4 -> PWM2signal5/1
  Demux/5 -> PWM2signal4/1
  pwm_inputs/1 -> Signal Specification/1
  Demux/6 -> PWM2signal6/1
  Demux/7 -> Terminator1/1
  Demux/8 -> Terminator2/1
  gyro_meas/1 -> Bus Creator meas/8  "omega_b_meas_radps"
  magne_meas/1 -> Terminator4/1
  press_alt_m/1 -> Bus Creator meas/6  "press_alt_m"
  gps_pos/1 -> Selector2/1, Selector/1
  gps_speed/1 -> Bus Creator meas/14  "gps_speed"
  gps_velocity_ned/1 -> Bus Creator meas/10, Matrix Multiply2/2, Matrix Multiply1/2  "gps_vel_ned"
  runtime_usec/1 -> Terminator11/1
  Signal Specification/1 -> Demux/1
  PWM2signal6/1 -> Data Type Conversion5/1
  pitot_diff_pre/1 -> Bus Creator meas/5  "q_dyn_press"
  Selector/1 -> Bus Creator meas/3  "lat_long"
  Selector2/1 -> Bus Creator meas/4  "gps_alt"
  TAS_mps/1 -> Bus Creator meas/16  "TAS_mps"
  Transpose/1 -> Matrix Multiply1/1
  Ground1/1 -> Bus Creator meas/11  "V_b_meas"
  Ground2/1 -> Bus Creator meas/12  "V_yaw"
  Ground/1 -> Bus Creator meas/9  "spare"
  Matrix Multiply1/1 -> Terminator/1  "V_b_meas"
  Matrix Multiply2/1 -> Terminator3/1  "V_yaw"
  Data Type Conversion/1 -> Left_up/1
  Data Type Conversion1/1 -> Left_side/1
  Data Type Conversion2/1 -> Right_up/1
  Data Type Conversion3/1 -> Right_side/1
  Data Type Conversion4/1 -> radio_switch/1
  Data Type Conversion5/1 -> radio_siwtch2/1

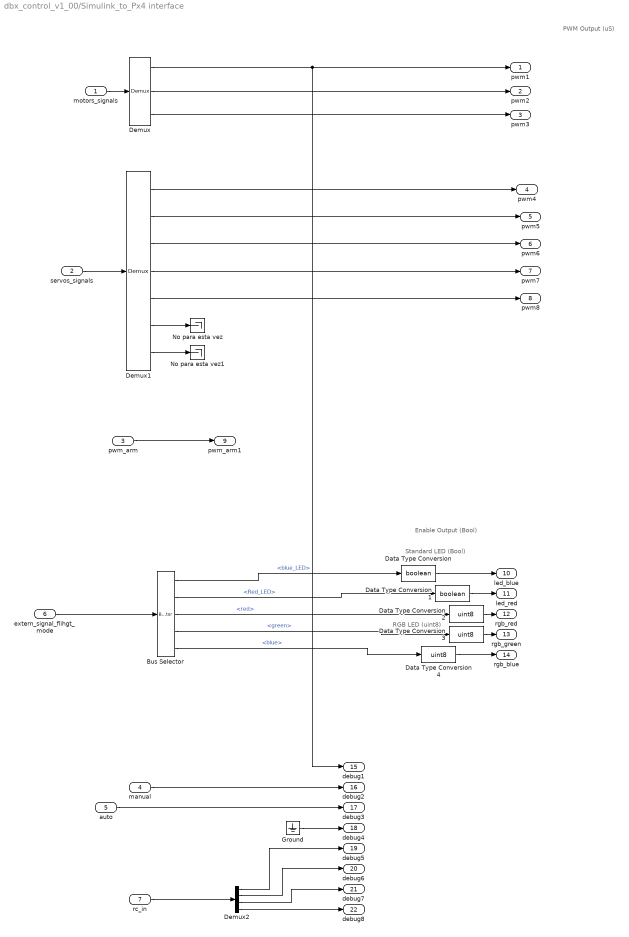
== system dbx_control_v1_00/Simulink_to_Px4 interface ==
  note: RGB LED (uint8)
  note: Standard LED (Bool)
  note: PWM Output (uS)
  note: Enable Output (Bool)
  motors_signals : Inport
  servos_signals : Inport  Port=2
  pwm_arm : Inport  Port=3
  manual : Inport  Port=4
  auto : Inport  Port=5
  extern_signal_flihgt_mode : Inport  Port=6
  rc_in : Inport  Port=7
  Bus Selector : BusSelector  OutputSignals=blue_LED,Red_LED,RGBLED.red,RGBLED.green,RGBLED.blue
  Data Type Conversion : DataTypeConversion  OutDataTypeStr=boolean
  Data Type Conversion1 : DataTypeConversion  OutDataTypeStr=boolean
  Data Type Conversion2 : DataTypeConversion  OutDataTypeStr=uint8
  Data Type Conversion3 : DataTypeConversion  OutDataTypeStr=uint8
  Data Type Conversion4 : DataTypeConversion  OutDataTypeStr=uint8
  Demux : Demux  Outputs=3
  Demux1 : Demux  Outputs=7
  Demux2 : Demux
  Ground : Ground
  No para esta vez : Terminator
  No para esta vez1 : Terminator
  pwm1 : Outport  PortDimensions=1  SampleTime=T_ctrl
  pwm2 : Outport  Port=2  PortDimensions=1  SampleTime=T_ctrl
  pwm3 : Outport  Port=3  PortDimensions=1  SampleTime=T_ctrl
  pwm4 : Outport  Port=4  PortDimensions=1  SampleTime=T_ctrl
  pwm5 : Outport  Port=5  PortDimensions=1  SampleTime=T_ctrl
  pwm6 : Outport  Port=6  PortDimensions=1  SampleTime=T_ctrl
  pwm7 : Outport  Port=7  PortDimensions=1  SampleTime=T_ctrl
  pwm8 : Outport  Port=8  PortDimensions=1  SampleTime=T_ctrl
  pwm_arm1 : Outport  Port=9  PortDimensions=1  SampleTime=T_ctrl
  led_blue : Outport  Port=10  OutDataTypeStr=boolean  PortDimensions=1  SampleTime=T_ctrl
  led_red : Outport  Port=11  OutDataTypeStr=boolean  PortDimensions=1  SampleTime=T_ctrl
  rgb_red : Outport  Port=12  OutDataTypeStr=uint8  PortDimensions=1  SampleTime=T_ctrl
  rgb_green : Outport  Port=13  OutDataTypeStr=uint8  PortDimensions=1  SampleTime=T_ctrl
  rgb_blue : Outport  Port=14  OutDataTypeStr=uint8  PortDimensions=1  SampleTime=T_ctrl
  debug1 : Outport  Port=15  PortDimensions=1  SampleTime=T_ctrl
  debug2 : Outport  Port=16  PortDimensions=1  SampleTime=T_ctrl
  debug3 : Outport  Port=17  PortDimensions=1  SampleTime=T_ctrl
  debug4 : Outport  Port=18  PortDimensions=1  SampleTime=T_ctrl
  debug5 : Outport  Port=19  PortDimensions=1  SampleTime=T_ctrl
  debug6 : Outport  Port=20  PortDimensions=1  SampleTime=T_ctrl
  debug7 : Outport  Port=21  PortDimensions=1  SampleTime=T_ctrl
  debug8 : Outport  Port=22  PortDimensions=1  SampleTime=T_ctrl
  wires:
  extern_signal_flihgt_mode/1 -> Bus Selector/1
  Bus Selector/2 -> Data Type Conversion1/1  "<Red_LED>"
  pwm_arm/1 -> pwm_arm1/1
  Bus Selector/3 -> Data Type Conversion2/1  "<red>"
  Bus Selector/4 -> Data Type Conversion3/1  "<green>"
  Bus Selector/5 -> Data Type Conversion4/1  "<blue>"
  Data Type Conversion/1 -> led_blue/1
  Data Type Conversion1/1 -> led_red/1
  Data Type Conversion2/1 -> rgb_red/1
  Data Type Conversion3/1 -> rgb_green/1
  Data Type Conversion4/1 -> rgb_blue/1
  Bus Selector/1 -> Data Type Conversion/1  "<blue_LED>"
  motors_signals/1 -> Demux/1
  Demux/1 -> debug1/1, pwm1/1
  Demux/2 -> pwm2/1
  servos_signals/1 -> Demux1/1
  rc_in/1 -> Demux2/1
  manual/1 -> debug2/1
  auto/1 -> debug3/1
  Demux2/4 -> debug8/1
  Demux2/3 -> debug7/1
  Demux2/2 -> debug6/1
  Demux2/1 -> debug5/1
  Ground/1 -> debug4/1
  Demux/3 -> pwm3/1
  Demux1/1 -> pwm4/1
  Demux1/2 -> pwm5/1
  Demux1/3 -> pwm6/1
  Demux1/4 -> pwm7/1
  Demux1/5 -> pwm8/1
  Demux1/6 -> No para esta vez/1
  Demux1/7 -> No para esta vez1/1

== system dbx_control_v1_00/Status signals ==
  manual : Inport
  auto : Inport  Port=2
  pwm_arm : Inport  Port=3
  Ground1 : Ground
  Logical Operator1 : Logic  Operator=NOT  IconShape=distinctive  AllPortsSameDT=off  OutDataTypeStr=boolean
  Beep : Outport
  Red_LED : Outport  Port=2
  blue_LED : Outport  Port=3
  blue_RGBLED : Outport  Port=4
  Red_RGBLED : Outport  Port=5
  green_RGBLED : Outport  Port=6
  wires:
  Ground1/1 -> Beep/1
  manual/1 -> Red_RGBLED/1, Red_LED/1
  auto/1 -> blue_RGBLED/1, blue_LED/1
  pwm_arm/1 -> Logical Operator1/1
  Logical Operator1/1 -> green_RGBLED/1

== system dbx_control_v1_00/Auto-mode autopiloto/Activation bus ==
  Activation : Inport
  Activation1 : Inport  Port=2
  Activation2 : Inport  Port=3
  Activation3 : Inport  Port=4
  Bus Creator : BusCreator  Inputs=6
  Ground : Ground
  Ground1 : Ground
  Activation bus : Outport
  wires:
  Ground1/1 -> Bus Creator/2  "alt_act"
  Activation/1 -> Bus Creator/3  "vel_yaw_xy_act"
  Activation2/1 -> Bus Creator/5  "euler_act"
  Activation3/1 -> Bus Creator/6  "b_rates_act"
  Bus Creator/1 -> Activation bus/1
  Ground/1 -> Bus Creator/1  "pos_xy_act"
  Activation1/1 -> Bus Creator/4  "vel_yaw_z_act"

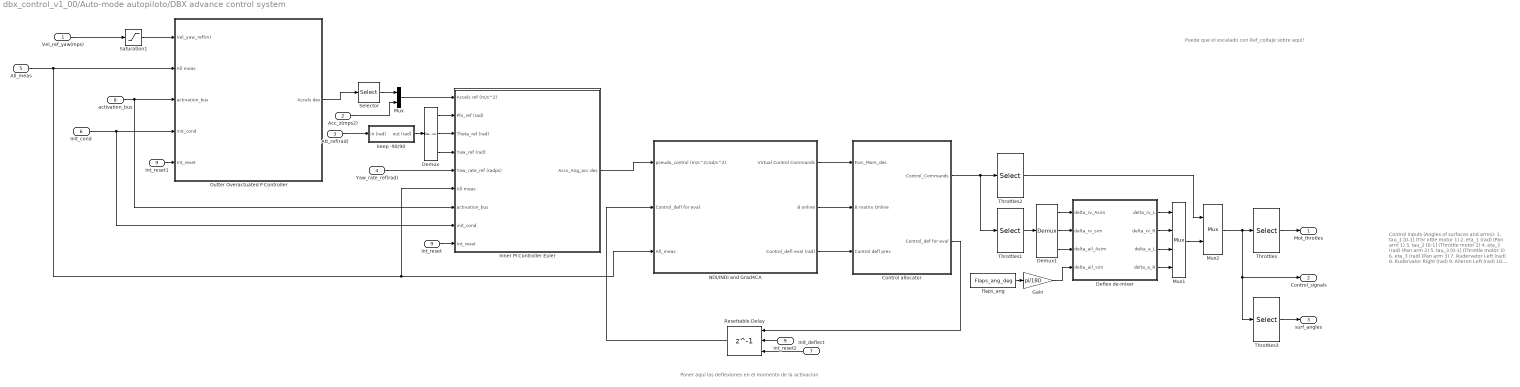
== system dbx_control_v1_00/Auto-mode autopiloto/DBX advance control system ==
  note: Puede que el escalado con Ref_coltaje sobre aqui!
  note: Poner aqui las deflexiones en el momento de la activacion
  note: Control inputs (Angles  of surfaces and arms):
      |
      | 1. tau_1 [0-1] (Thr ottle motor 1)
      | 2. eta_1 (rad)  (Pan arm 1)
      |
      | 3. tau_2 [0-1] (Throttle motor 2)
      | 4. eta_2 (rad)  (Pan arm 2)
      |
      | 5. tau_3 [0-1] (Throttle motor 3)
      | 6. eta_3 (rad)  (Pan arm  3)
      |
      | 7. Rudervator Left (rad)
      | 8. Rudervator Right (rad)
      | 9. Aileron Left (rad)
      | 10. Aielron Right (rad)
  Vel_ref_yaw(mps) : Inport
  Acc_z(mps2) : Inport  Port=2
  Att_ref(rad) : Inport  Port=3
  Yaw_rate_ref(rad) : Inport  Port=4
  All_meas : Inport  Port=5
  Init_cond : Inport  Port=6
  Init_deflect : Inport  Port=7  PortDimensions=[9,1]
  activation_bus : Inport  Port=8
  Int_reset : Inport  Port=9
  Control allocator : Subsystem  RTWFcnName=abc  RTWFileName=asas  VariantControl=Control Allocator: NO RECONFIG
      settings: MinAlgLoopOccurrences=on  RTWFcnNameOpts=User specified  RTWFileNameOpts=User specified
  Deflex de-mixer : Subsystem  TreatAsAtomicUnit=on
  Demux : Demux  Outputs=3
  Demux1 : Demux  Outputs=3
  Gain : Gain  Gain=pi/180
  Inner PI Controller Euler : Subsystem  VariantControl=PI_quat
  Int_reset1 : InportShadow  Port=9
  Int_reset2 : InportShadow  Port=9
  Mux : Mux  Inputs=[2,1]
  Mux1 : Mux
  Mux2 : Mux  Inputs=[6,4]
  NDI/INDI and Grad4CA : Subsystem  Variant=on  VariantControl=NDI: NO RECONFIG  OverrideUsingVariant=NDI_incremental_grad
  Outter Overactuated P Controller : Subsystem  VariantControl=Overactuated P Controller
  Resettable Delay : Delay  DelayLength=1  InitialConditionSource=Input port  ExternalReset=Either  InputProcessing=Inherited  SampleTime=T_ctrl
      settings: InputPortMap=u0,r5,p4
  Saturation1 : Saturate  UpperLimit=[10,10,v_i0]'  LowerLimit=-[10,10,2*v_i0]'
  Selector : Selector  InputPortWidth=3  Indices=1:2
  Throttles : Selector  InputPortWidth=10  Indices=[1,3,5]
  Throttles1 : Selector  InputPortWidth=9  Indices=[7:9]
  Throttles2 : Selector  InputPortWidth=9  Indices=[1:6]
  Throttles3 : Selector  InputPortWidth=10  Indices=[2,4,6,7,8,9,10]
  flaps_ang : Constant  Value=Flaps_ang_deg  OutDataTypeStr=single
  keep -90/90 : Subsystem
  Mot_throtles : Outport
  Control_signals : Outport  Port=2
  surf_angles : Outport  Port=3
  wires:
  All_meas/1 -> Inner PI Controller Euler/6(All meas), NDI/INDI and Grad4CA/3(All_meas), Outter Overactuated P Controller/2(All meas)
  NDI/INDI and Grad4CA/3(Control_defl eval (rad)) -> Control allocator/3(Control defl prev)
  keep -90/90/1(out (rad)) -> Demux/1
  Demux/3 -> Inner PI Controller Euler/4(Yaw_ref (rad))
  Demux/2 -> Inner PI Controller Euler/3(Theta_ref (rad))
  Demux/1 -> Inner PI Controller Euler/2(Phi_ref (rad))
  Att_ref(rad)/1 -> keep -90/90/1(in (rad))
  Throttles/1 -> Mot_throtles/1
  Control allocator/1(Control_Commands) -> Throttles1/1, Throttles2/1
  Resettable Delay/1 -> NDI/INDI and Grad4CA/2(Control_defl for eval)
  Vel_ref_yaw(mps)/1 -> Saturation1/1
  Saturation1/1 -> Outter Overactuated P Controller/1(Vel_yaw_ref(m))
  Init_cond/1 -> Inner PI Controller Euler/8(init_cond), Outter Overactuated P Controller/4(init_cond)
  activation_bus/1 -> Inner PI Controller Euler/7(activation_bus), Outter Overactuated P Controller/3(activation_bus)
  Control allocator/2(Control_def for eval) -> Resettable Delay/1
  NDI/INDI and Grad4CA/2(B online) -> Control allocator/2(B matrix Online)
  Inner PI Controller Euler/1(Accs_Ang_acc des) -> NDI/INDI and Grad4CA/1(pseudo_control (m/s^2;rad/s^2))
  Demux1/2 -> Deflex de-mixer/2(delta_rv_sim)
  Demux1/3 -> Deflex de-mixer/3(delta_ail_Asim)
  Demux1/1 -> Deflex de-mixer/1(delta_rv_Asim)
  Throttles1/1 -> Demux1/1
  Throttles2/1 -> Mux2/1
  Deflex de-mixer/1(delta_rv_L) -> Mux1/1
  Deflex de-mixer/2(delta_rv_R) -> Mux1/2
  Deflex de-mixer/3(delta_a_L) -> Mux1/3
  Deflex de-mixer/4(delta_a_R) -> Mux1/4
  Mux1/1 -> Mux2/2
  Mux2/1 -> Throttles3/1, Control_signals/1, Throttles/1
  Throttles3/1 -> surf_angles/1
  Yaw_rate_ref(rad)/1 -> Inner PI Controller Euler/5(Yaw_rate_ref (radps))
  Int_reset/1 -> Inner PI Controller Euler/9(Int_reset)
  Int_reset1/1 -> Outter Overactuated P Controller/5(Int_reset)
  Acc_z(mps2)/1 -> Mux/2
  Init_deflect/1 -> Resettable Delay/3
  Int_reset2/1 -> Resettable Delay/2
  NDI/INDI and Grad4CA/1(Virtual Control Commands) -> Control allocator/1(Forc_Mom_des)
  Selector/1 -> Mux/1
  flaps_ang/1 -> Gain/1
  Gain/1 -> Deflex de-mixer/4(delta_ail_sim)
  Outter Overactuated P Controller/1(Accels des) -> Selector/1
  Mux/1 -> Inner PI Controller Euler/1(Accels ref (m/s^2))
